simulink model "Simple_4Quad_payload_04"  (R2018b)
settings: Solver=VariableStepAuto  StartTime=0.0  StopTime=60  RelTol=1e-3
InitFcn:
  | Simple_4Quad_payload_04_const
values from neighbouring files (symbols this model uses):
  All_rho = [d1 0 0 ... (first row only)    [Colab_4Quad_model_01_const.m]    (also in Colab_4Quad_model_02_const.m; Simple_4Quad_payload_04_const.m; Simple_4Quad_payload_05_const.m; Simple_4Quad_payload_06_const.m)
  B_ob = [zeros(3);eye(3)]    [Simple_4Quad_payload_04_const.m]    (also in Simple_4Quad_payload_05_const.m; Simple_4Quad_payload_06_const.m; Simple_4Quad_payload_07_const.m; Simple_4Quad_payload_08_const.m)
  BBT_inv = ((B'*B)^(-1))*B'    [Simple_2Quad_payload_03_const.m]    (also in Simple_4Quad_payload_04_const.m = ((BR'*BR)^(-1))*BR'; Simple_4Quad_payload_05_const.m = ((BR'*BR)^(-1))*BR'; Simple_4Quad_payload_06_const.m = ((BR'*BR)^(-1))*BR'; Simple_4Quad_payload_07_const.m = ((BR'*BR)^(-1))*BR')
  BR = 1e0*eye(n)    [Simple_4Quad_payload_04_const.m]    (also in Simple_4Quad_payload_05_const.m; Simple_4Quad_payload_06_const.m; Simple_4Quad_payload_07_const.m; Simple_4Quad_payload_08_const.m)
  C_ob = [eye(3) zeros(3)]    [Simple_4Quad_payload_04_const.m]    (also in Simple_4Quad_payload_05_const.m; Simple_4Quad_payload_06_const.m; Simple_4Quad_payload_07_const.m; Simple_4Quad_payload_08_const.m)
  d1 = 0.25    [Colab_4Quad_model_01_const.m]    (also in Colab_4Quad_model_02_const.m = 0.5; Simple_4Quad_payload_01_const.m = 1; Simple_4Quad_payload_02_const.m = 1; Simple_4Quad_payload_03_const.m = 1)
  d2 = 0.25    [Colab_4Quad_model_01_const.m]    (also in Colab_4Quad_model_02_const.m = 0.5; Simple_4Quad_payload_01_const.m = 1; Simple_4Quad_payload_02_const.m = 1; Simple_4Quad_payload_03_const.m = 1)
  Des_rel_dist = 2    [Simple_4Quad_payload_01_const.m]    (also in Simple_4Quad_payload_02_const.m = 4; Simple_4Quad_payload_03_const.m = 4; Simple_4Quad_payload_04_const.m; Simple_4Quad_payload_05_const.m)
  g = 9.81    [Colab_4Quad_model_01_const.m]    (also in Colab_4Quad_model_02_const.m; Simple_2Quad_payload_01_const.m; Simple_2Quad_payload_02_const.m; Simple_2Quad_payload_03_const.m)
  gamma_0 = 1e-0*diag([1e-3;1e-0])    [Simple_2Quad_payload_03_const.m]    (also in Simple_4Quad_payload_04_const.m = 1e-0*diag([1e-6*ones(3,1);1e-0*ones(3,1)]); Simple_4Quad_payload_05_const.m = 1e-1*diag([1e-6*ones(3,1);1e-0*ones(3,1)]); Simple_4Quad_payload_06_const.m = 1e-0*diag([1e-6*ones(3,1);1e-0*ones(3,1)]); Simple_4Quad_payload_07_const.m = 1e-0*diag([1e-6*ones(3,1);1e-0*ones(3,1)]))
  gamma_1 = 1e+2*diag([1e-3;1e-0])    [Simple_2Quad_payload_03_const.m]    (also in Simple_4Quad_payload_04_const.m = 1e+2*diag([1e-6*ones(3,1);1e-0*ones(3,1)]); Simple_4Quad_payload_05_const.m = 1e+2*diag([1e-6*ones(3,1);1e-0*ones(3,1)]); Simple_4Quad_payload_06_const.m = 1e+3*diag([1e-6*ones(3,1);1e-0*ones(3,1)]); Simple_4Quad_payload_07_const.m = 1e+3*diag([1e-6*ones(3,1);1e-0*ones(3,1)]))
  Ix = 0.166667    [Colab_4Quad_model_01_const.m]    (also in Colab_4Quad_model_02_const.m = 0.02; Simple_4Quad_payload_01_const.m = 1; Simple_4Quad_payload_02_const.m = 1; Simple_4Quad_payload_03_const.m = 1)
  Iy = 0.166667    [Colab_4Quad_model_01_const.m]    (also in Colab_4Quad_model_02_const.m = 0.02; Simple_4Quad_payload_01_const.m = 1; Simple_4Quad_payload_02_const.m = 1; Simple_4Quad_payload_03_const.m = 1)
  Iz = 0.166667    [Colab_4Quad_model_01_const.m]    (also in Colab_4Quad_model_02_const.m = 0.02; Simple_4Quad_payload_01_const.m = 1; Simple_4Quad_payload_02_const.m = 1; Simple_4Quad_payload_03_const.m = 1)
  Jo = diag([Ix;Iy;Iz])    [Colab_4Quad_model_01_const.m]    (also in Colab_4Quad_model_02_const.m; Simple_4Quad_payload_04_const.m; Simple_4Quad_payload_05_const.m; Simple_4Quad_payload_06_const.m)
  Jq = diag([0.0291 0.0291 0.0552])    [Colab_4Quad_model_01_const.m]    (also in Colab_4Quad_model_02_const.m = diag([0.03 0.03 0.06]); Simple_4Quad_payload_03_const.m = 1.2416e-3 * diag([1 1 2]); Simple_4Quad_payload_04_const.m = 1 * diag([1 1 2]); Simple_4Quad_payload_05_const.m = 1 * diag([1 1 2]))
  k1 = 1    [Simple_2Quad_payload_03_const.m]    (also in Simple_4Quad_payload_04_const.m; Simple_4Quad_payload_05_const.m; Simple_4Quad_payload_06_const.m; Simple_4Quad_payload_07_const.m)
  k2 = 0.1    [Simple_2Quad_payload_03_const.m]    (also in Simple_4Quad_payload_04_const.m; Simple_4Quad_payload_05_const.m; Simple_4Quad_payload_06_const.m; Simple_4Quad_payload_07_const.m)
  ki1_N = 0    [Simple_4Quad_payload_02_const.m]    (also in Simple_4Quad_payload_03_const.m; Simple_4Quad_payload_04_const.m; Simple_4Quad_payload_05_const.m; Simple_4Quad_payload_06_const.m)
  ki1_S = 0    [Simple_4Quad_payload_02_const.m]    (also in Simple_4Quad_payload_03_const.m; Simple_4Quad_payload_04_const.m)
  ki2_N = 0    [Simple_4Quad_payload_02_const.m]    (also in Simple_4Quad_payload_03_const.m; Simple_4Quad_payload_04_const.m; Simple_4Quad_payload_05_const.m; Simple_4Quad_payload_06_const.m = 10)
  ki2_S = 0    [Simple_4Quad_payload_02_const.m]    (also in Simple_4Quad_payload_03_const.m; Simple_4Quad_payload_04_const.m)
  kp1_N = 10    [Simple_4Quad_payload_02_const.m]    (also in Simple_4Quad_payload_03_const.m; Simple_4Quad_payload_04_const.m; Simple_4Quad_payload_05_const.m = 1; Simple_4Quad_payload_06_const.m = 1)
  kp1_S = 10    [Simple_4Quad_payload_02_const.m]    (also in Simple_4Quad_payload_03_const.m; Simple_4Quad_payload_04_const.m)
  kp2_N = 100    [Simple_4Quad_payload_02_const.m]    (also in Simple_4Quad_payload_03_const.m; Simple_4Quad_payload_04_const.m; Simple_4Quad_payload_05_const.m = 1; Simple_4Quad_payload_06_const.m = 1)
  kp2_S = 100    [Simple_4Quad_payload_02_const.m]    (also in Simple_4Quad_payload_03_const.m; Simple_4Quad_payload_04_const.m)
  l = 3.1819    [Colab_4Quad_model_01_const.m]    (also in Colab_4Quad_model_02_const.m = 3; Simple_2Quad_payload_04_const.m = 1; Simple_4Quad_payload_01_const.m = 1; Simple_4Quad_payload_02_const.m = 2)
  m = 1.5    [Colab_4Quad_model_01_const.m]    (also in Colab_4Quad_model_02_const.m; Simple_2Quad_payload_04_const.m = 1; Simple_4Quad_payload_01_const.m = 1; Simple_4Quad_payload_02_const.m = 1)
  M = 1.0    (= 1)    [Colab_4Quad_model_01_const.m]    (also in Colab_4Quad_model_02_const.m; Simple_2Quad_payload_01_const.m; Simple_2Quad_payload_02_const.m; Simple_2Quad_payload_03_const.m)
  Md = 1*[1;1;1]    [Simple_2Quad_payload_04_const.m]    (also in Simple_4Quad_payload_01_const.m = 1*[1;1;1;1;1;1]; Simple_4Quad_payload_02_const.m = 1*[1;1;1;1;1;1]; Simple_4Quad_payload_03_const.m = 1*[1;1;1;1;1;1]; Simple_4Quad_payload_04_const.m = 1*[1;1;1;1;1;1])
  n = 2    [Simple_2Quad_payload_03_const.m]    (also in Simple_4Quad_payload_03_const.m = 6; Simple_4Quad_payload_04_const.m = 6; Simple_4Quad_payload_05_const.m = 6; Simple_4Quad_payload_06_const.m = 6)
  Q_ob = var_u_ob * eye(6)    [Simple_4Quad_payload_04_const.m]    (also in Simple_4Quad_payload_05_const.m; Simple_4Quad_payload_06_const.m; Simple_4Quad_payload_07_const.m; Simple_4Quad_payload_08_const.m)
  QR = 1e-0*eye(n)    [Simple_4Quad_payload_04_const.m]    (also in Simple_4Quad_payload_05_const.m = 1e-1*eye(n); Simple_4Quad_payload_06_const.m; Simple_4Quad_payload_07_const.m; Simple_4Quad_payload_08_const.m)
  R = 1e+0*eye(n)    [Simple_2Quad_payload_03_const.m]    (also in Simple_4Quad_payload_04_const.m = 1e+0*eye(m); Simple_4Quad_payload_05_const.m = 1e+0*eye(m); Simple_4Quad_payload_06_const.m; Simple_4Quad_payload_07_const.m)
  R_ob = var_y_ob * eye(3)    [Simple_4Quad_payload_04_const.m]    (also in Simple_4Quad_payload_05_const.m; Simple_4Quad_payload_06_const.m; Simple_4Quad_payload_07_const.m; Simple_4Quad_payload_08_const.m)
  rho_0 = 1e-0    (= 1)    [Simple_2Quad_payload_03_const.m]    (also in Simple_4Quad_payload_04_const.m; Simple_4Quad_payload_05_const.m = 0.1; Simple_4Quad_payload_06_const.m; Simple_4Quad_payload_07_const.m)
  rho_1 = 1e-0    (= 1)    [Simple_2Quad_payload_03_const.m]    (also in Simple_4Quad_payload_04_const.m; Simple_4Quad_payload_05_const.m; Simple_4Quad_payload_06_const.m; Simple_4Quad_payload_07_const.m)
libraries: simulink x16
(part 3 of 4)

== system Simple_4Quad_payload_04/Controllers and Observers/Cotnroller and Observer - Agent1 /PID_alpha1 ==
  alpha1_des : Inport
  alpha1 : Inport  Port=2
  D_alpha1 : Inport  Port=3
  PID Controller : simulink/Continuous/PID Controller  Controller=PID  Form=Parallel  TimeDomain=Continuous-time  SampleTime=-1  IntegratorMethod=Forward Euler  FilterMethod=Forward Euler  ControllerParametersSource=internal  P=kp1_N  I=ki1_N  D=0  UseFilter=on  N=100  TunerSelectOption=Transfer Function Based (PID Tuner App)  InitialConditionSource=internal  InitialConditionForIntegrator=0  InitialConditionForFilter=0  DifferentiatorICPrevScaledInput=0  ExternalReset=none  TrackingMode=off  Kt=1  LimitOutput=off  UpperSaturationLimit=inf  LowerSaturationLimit=-inf  LinearizeAsGain=on  AntiWindupMode=none  Kb=1  POutMin=[]  POutMax=[]  IOutMin=[]  IOutMax=[]  DOutMin=[]  DOutMax=[]  NOutMin=[]  NOutMax=[]  SumOutMin=[]  SumOutMax=[]  SaturationOutMin=[]  SaturationOutMax=[]  PParamMin=[]  PParamMax=[]  IParamMin=[]  IParamMax=[]  DParamMin=[]  DParamMax=[]  NParamMin=[]  NParamMax=[]  KbParamMin=[]  KbParamMax=[]  KtParamMin=[]  KtParamMax=[]  KbOutMin=[]  KbOutMax=[]  KtOutMin=[]  KtOutMax=[]  IntegratorOutMin=[]  IntegratorOutMax=[]  FilterOutMin=[]  FilterOutMax=[]  SumI1OutMin=[]  SumI1OutMax=[]  SumI2OutMin=[]  SumI2OutMax=[]  SumI3OutMin=[]  SumI3OutMax=[]  SumI4OutMin=[]  SumI4OutMax=[]  SumDOutMin=[]  SumDOutMax=[]  DifferentiatorOutMin=[]  DifferentiatorOutMax=[]  FilterDiffOutCoefMin=[]  FilterDiffOutCoefMax=[]  ReciprocalOutMin=[]  ReciprocalOutMax=[]  SumDenOutMin=[]  SumDenOutMax=[]  SumNumOutMin=[]  SumNumOutMax=[]  DivideOutMin=[]  DivideOutMax=[]  IntegratorContinuousStateAttributes=''  IntegratorStateMustResolveToSignalObject=off  IntegratorRTWStateStorageClass=Auto  FilterContinuousStateAttributes=''  FilterStateMustResolveToSignalObject=off  FilterRTWStateStorageClass=Auto  ParallelPVariant=InternalParameters  IdealPVariant=Disabled  IVariant=InternalParameters  DVariant=InternalParameters  IntegratorVariant=Continuous  SatVariant=Disabled  AWVariant=Passthrough  PCopyVariant=Disabled  TRVariant=Disabled  FdbkBlocksVariant=Forward  IdealPFdbkVariant=Disabled  SatFdbkVariant=Disabled  DerivativeFilterVariant=ContFilter  NVariant=InternalParameters  NCopyVariant=Disabled  FilterICVariant=InternalICsFilter  IntegratorICVariant=InternalICs  ExternalResetVariant=Disabled  TRSumVariant=Passthrough  SumFdbkVariant=Disabled  SumVariant=Sum_PID
  PID Controller1 : simulink/Continuous/PID Controller  Controller=PID  Form=Parallel  TimeDomain=Continuous-time  SampleTime=-1  IntegratorMethod=Forward Euler  FilterMethod=Forward Euler  ControllerParametersSource=internal  P=kp2_N  I=ki2_N  D=0  UseFilter=on  N=100  TunerSelectOption=Transfer Function Based (PID Tuner App)  InitialConditionSource=internal  InitialConditionForIntegrator=0  InitialConditionForFilter=0  DifferentiatorICPrevScaledInput=0  ExternalReset=none  TrackingMode=off  Kt=1  LimitOutput=off  UpperSaturationLimit=inf  LowerSaturationLimit=-inf  LinearizeAsGain=on  AntiWindupMode=none  Kb=1  POutMin=[]  POutMax=[]  IOutMin=[]  IOutMax=[]  DOutMin=[]  DOutMax=[]  NOutMin=[]  NOutMax=[]  SumOutMin=[]  SumOutMax=[]  SaturationOutMin=[]  SaturationOutMax=[]  PParamMin=[]  PParamMax=[]  IParamMin=[]  IParamMax=[]  DParamMin=[]  DParamMax=[]  NParamMin=[]  NParamMax=[]  KbParamMin=[]  KbParamMax=[]  KtParamMin=[]  KtParamMax=[]  KbOutMin=[]  KbOutMax=[]  KtOutMin=[]  KtOutMax=[]  IntegratorOutMin=[]  IntegratorOutMax=[]  FilterOutMin=[]  FilterOutMax=[]  SumI1OutMin=[]  SumI1OutMax=[]  SumI2OutMin=[]  SumI2OutMax=[]  SumI3OutMin=[]  SumI3OutMax=[]  SumI4OutMin=[]  SumI4OutMax=[]  SumDOutMin=[]  SumDOutMax=[]  DifferentiatorOutMin=[]  DifferentiatorOutMax=[]  FilterDiffOutCoefMin=[]  FilterDiffOutCoefMax=[]  ReciprocalOutMin=[]  ReciprocalOutMax=[]  SumDenOutMin=[]  SumDenOutMax=[]  SumNumOutMin=[]  SumNumOutMax=[]  DivideOutMin=[]  DivideOutMax=[]  IntegratorContinuousStateAttributes=''  IntegratorStateMustResolveToSignalObject=off  IntegratorRTWStateStorageClass=Auto  FilterContinuousStateAttributes=''  FilterStateMustResolveToSignalObject=off  FilterRTWStateStorageClass=Auto  ParallelPVariant=InternalParameters  IdealPVariant=Disabled  IVariant=InternalParameters  DVariant=InternalParameters  IntegratorVariant=Continuous  SatVariant=Disabled  AWVariant=Passthrough  PCopyVariant=Disabled  TRVariant=Disabled  FdbkBlocksVariant=Forward  IdealPFdbkVariant=Disabled  SatFdbkVariant=Disabled  DerivativeFilterVariant=ContFilter  NVariant=InternalParameters  NCopyVariant=Disabled  FilterICVariant=InternalICsFilter  IntegratorICVariant=InternalICs  ExternalResetVariant=Disabled  TRSumVariant=Passthrough  SumFdbkVariant=Disabled  SumVariant=Sum_PID
  Scope3 : Scope  NumInputPorts=3
  Sum : Sum  Inputs=|+-
  Sum1 : Sum  Inputs=|+-
  N1 : Outport
  wires:
  D_alpha1/1 -> Sum1/2
  alpha1/1 -> Sum/2
  alpha1_des/1 -> Sum/1
  Sum1/1 -> Scope3/2, PID Controller1/1
  Sum/1 -> PID Controller/1, Scope3/1
  PID Controller1/1 -> Scope3/3, N1/1
  PID Controller/1 -> Sum1/1

== system Simple_4Quad_payload_04/Controllers and Observers/Cotnroller and Observer - Agent1 /PID_beta1 ==
  beta1_des : Inport
  beta1 : Inport  Port=2
  D_beta1 : Inport  Port=3
  PID Controller : simulink/Continuous/PID Controller  Controller=PID  Form=Parallel  TimeDomain=Continuous-time  SampleTime=-1  IntegratorMethod=Forward Euler  FilterMethod=Forward Euler  ControllerParametersSource=internal  P=kp1_S  I=ki1_S  D=0  UseFilter=on  N=100  TunerSelectOption=Transfer Function Based (PID Tuner App)  InitialConditionSource=internal  InitialConditionForIntegrator=0  InitialConditionForFilter=0  DifferentiatorICPrevScaledInput=0  ExternalReset=none  TrackingMode=off  Kt=1  LimitOutput=off  UpperSaturationLimit=inf  LowerSaturationLimit=-inf  LinearizeAsGain=on  AntiWindupMode=none  Kb=1  POutMin=[]  POutMax=[]  IOutMin=[]  IOutMax=[]  DOutMin=[]  DOutMax=[]  NOutMin=[]  NOutMax=[]  SumOutMin=[]  SumOutMax=[]  SaturationOutMin=[]  SaturationOutMax=[]  PParamMin=[]  PParamMax=[]  IParamMin=[]  IParamMax=[]  DParamMin=[]  DParamMax=[]  NParamMin=[]  NParamMax=[]  KbParamMin=[]  KbParamMax=[]  KtParamMin=[]  KtParamMax=[]  KbOutMin=[]  KbOutMax=[]  KtOutMin=[]  KtOutMax=[]  IntegratorOutMin=[]  IntegratorOutMax=[]  FilterOutMin=[]  FilterOutMax=[]  SumI1OutMin=[]  SumI1OutMax=[]  SumI2OutMin=[]  SumI2OutMax=[]  SumI3OutMin=[]  SumI3OutMax=[]  SumI4OutMin=[]  SumI4OutMax=[]  SumDOutMin=[]  SumDOutMax=[]  DifferentiatorOutMin=[]  DifferentiatorOutMax=[]  FilterDiffOutCoefMin=[]  FilterDiffOutCoefMax=[]  ReciprocalOutMin=[]  ReciprocalOutMax=[]  SumDenOutMin=[]  SumDenOutMax=[]  SumNumOutMin=[]  SumNumOutMax=[]  DivideOutMin=[]  DivideOutMax=[]  IntegratorContinuousStateAttributes=''  IntegratorStateMustResolveToSignalObject=off  IntegratorRTWStateStorageClass=Auto  FilterContinuousStateAttributes=''  FilterStateMustResolveToSignalObject=off  FilterRTWStateStorageClass=Auto  ParallelPVariant=InternalParameters  IdealPVariant=Disabled  IVariant=InternalParameters  DVariant=InternalParameters  IntegratorVariant=Continuous  SatVariant=Disabled  AWVariant=Passthrough  PCopyVariant=Disabled  TRVariant=Disabled  FdbkBlocksVariant=Forward  IdealPFdbkVariant=Disabled  SatFdbkVariant=Disabled  DerivativeFilterVariant=ContFilter  NVariant=InternalParameters  NCopyVariant=Disabled  FilterICVariant=InternalICsFilter  IntegratorICVariant=InternalICs  ExternalResetVariant=Disabled  TRSumVariant=Passthrough  SumFdbkVariant=Disabled  SumVariant=Sum_PID
  PID Controller1 : simulink/Continuous/PID Controller  Controller=PID  Form=Parallel  TimeDomain=Continuous-time  SampleTime=-1  IntegratorMethod=Forward Euler  FilterMethod=Forward Euler  ControllerParametersSource=internal  P=kp2_S  I=ki2_S  D=0  UseFilter=on  N=100  TunerSelectOption=Transfer Function Based (PID Tuner App)  InitialConditionSource=internal  InitialConditionForIntegrator=0  InitialConditionForFilter=0  DifferentiatorICPrevScaledInput=0  ExternalReset=none  TrackingMode=off  Kt=1  LimitOutput=off  UpperSaturationLimit=inf  LowerSaturationLimit=-inf  LinearizeAsGain=on  AntiWindupMode=none  Kb=1  POutMin=[]  POutMax=[]  IOutMin=[]  IOutMax=[]  DOutMin=[]  DOutMax=[]  NOutMin=[]  NOutMax=[]  SumOutMin=[]  SumOutMax=[]  SaturationOutMin=[]  SaturationOutMax=[]  PParamMin=[]  PParamMax=[]  IParamMin=[]  IParamMax=[]  DParamMin=[]  DParamMax=[]  NParamMin=[]  NParamMax=[]  KbParamMin=[]  KbParamMax=[]  KtParamMin=[]  KtParamMax=[]  KbOutMin=[]  KbOutMax=[]  KtOutMin=[]  KtOutMax=[]  IntegratorOutMin=[]  IntegratorOutMax=[]  FilterOutMin=[]  FilterOutMax=[]  SumI1OutMin=[]  SumI1OutMax=[]  SumI2OutMin=[]  SumI2OutMax=[]  SumI3OutMin=[]  SumI3OutMax=[]  SumI4OutMin=[]  SumI4OutMax=[]  SumDOutMin=[]  SumDOutMax=[]  DifferentiatorOutMin=[]  DifferentiatorOutMax=[]  FilterDiffOutCoefMin=[]  FilterDiffOutCoefMax=[]  ReciprocalOutMin=[]  ReciprocalOutMax=[]  SumDenOutMin=[]  SumDenOutMax=[]  SumNumOutMin=[]  SumNumOutMax=[]  DivideOutMin=[]  DivideOutMax=[]  IntegratorContinuousStateAttributes=''  IntegratorStateMustResolveToSignalObject=off  IntegratorRTWStateStorageClass=Auto  FilterContinuousStateAttributes=''  FilterStateMustResolveToSignalObject=off  FilterRTWStateStorageClass=Auto  ParallelPVariant=InternalParameters  IdealPVariant=Disabled  IVariant=InternalParameters  DVariant=InternalParameters  IntegratorVariant=Continuous  SatVariant=Disabled  AWVariant=Passthrough  PCopyVariant=Disabled  TRVariant=Disabled  FdbkBlocksVariant=Forward  IdealPFdbkVariant=Disabled  SatFdbkVariant=Disabled  DerivativeFilterVariant=ContFilter  NVariant=InternalParameters  NCopyVariant=Disabled  FilterICVariant=InternalICsFilter  IntegratorICVariant=InternalICs  ExternalResetVariant=Disabled  TRSumVariant=Passthrough  SumFdbkVariant=Disabled  SumVariant=Sum_PID
  Scope3 : Scope  NumInputPorts=3
  Sum : Sum  Inputs=|+-
  Sum1 : Sum  Inputs=|+-
  S1 : Outport
  wires:
  D_beta1/1 -> Sum1/2
  PID Controller/1 -> Sum1/1
  PID Controller1/1 -> S1/1, Scope3/3
  Sum/1 -> Scope3/1, PID Controller/1
  Sum1/1 -> PID Controller1/1, Scope3/2
  beta1_des/1 -> Sum/1
  beta1/1 -> Sum/2

== system Simple_4Quad_payload_04/Controllers and Observers/Cotnroller and Observer - Agent1 /Rotation_Q1 ==
  Omega Q1 : Inport
  D Phi : MATLAB Function  TreatAsAtomicUnit=on
  Integrator : Integrator  InitialCondition=zeros(3,1)
  Mux : Mux  Inputs=2
  X_Rot_Q1 : Outport
  wires:
  D Phi/1(D_PHI_Q1) -> Integrator/1
  Omega Q1/1 -> D Phi/1(Omega_Q1), Mux/2
  Integrator/1 -> D Phi/2(PHI_Q1), Mux/1
  Mux/1 -> X_Rot_Q1/1

== system Simple_4Quad_payload_04/Controllers and Observers/Cotnroller and Observer - Agent1 /Rotational #1 ==
  x_rd : Inport
  X : Inport  Port=2
  CARE : MATLAB Function  TreatAsAtomicUnit=on
  Differentiator : Subsystem
  Integrator : Integrator  InitialCondition=zeros(n)
  Integrator1 : Integrator  InitialCondition=eye(n)
  Integrator2 : Integrator  InitialCondition=zeros(n,1)
  Integrator3 : Integrator  InitialCondition=zeros(n,1)
  Memory : Memory  InitialCondition=zeros(n,1)
  Sum : Sum  Inputs=|++
  g-Estimator : MATLAB Function  TreatAsAtomicUnit=on
  g-Estimator1 : MATLAB Function  TreatAsAtomicUnit=on
  main : MATLAB Function  TreatAsAtomicUnit=on
  output definition : MATLAB Function  TreatAsAtomicUnit=on
  variable change : MATLAB Function  TreatAsAtomicUnit=on
  ur1 : Outport
  tag scope: A_hat1_R=global, P1_R=global, e1_R=global, g_hat1_R=global
  wires:
  x_rd/1 -> variable change/2(Xd)
  X/1 -> variable change/1(X)
  CARE/1(DP) -> Integrator1/1
  Sum/1 -> main/1(sigma), g-Estimator/1(sigma), g-Estimator1/1(sigma)
  g-Estimator1/1(Da_hat) -> Integrator/1
  variable change/1(x_mod) -> main/7(x), g-Estimator1/2(x)
  Integrator1/1 -> g-Estimator1/3(P), CARE/1(P), [P1_R], g-Estimator/3(P), main/4(P)
  Integrator/1 -> [A_hat1_R], g-Estimator1/4(a_hat), CARE/2(a_hat), main/5(a_hat)
  g-Estimator/1(Dg_hat) -> Integrator2/1
  Differentiator/1(Dx_d) -> main/3(Dy_d)
  main/1(u) -> output definition/1(u), Memory/1
  Integrator3/1 -> main/2(zeta), Sum/1
  variable change/2(xd_mod) -> Differentiator/1(x_d)
  variable change/3(e_mod) -> [e1_R], Sum/2, Integrator3/1
  Memory/1 -> variable change/3(u)
  Integrator2/1 -> main/6(g_hat), [g_hat1_R], g-Estimator/2(g_hat)
  output definition/1(ur) -> ur1/1

== system Simple_4Quad_payload_04/Controllers and Observers/Controlelr and Observer - Agent3/Rotational #3/Differentiator ==
  x_d : Inport
  Integrator : Integrator  InitialCondition=zeros(n,1)
  Integrator1 : Integrator  InitialCondition=zeros(n,1)
  Scope : Scope
  Scope1 : Scope
  Sliding differentiator : MATLAB Function  TreatAsAtomicUnit=on
  Sliding differentiator1 : MATLAB Function  TreatAsAtomicUnit=on
  Sum : Sum  Inputs=|-+
  Dx_d : Outport
  wires:
  Integrator1/1 -> Sum/2
  Sum/1 -> Sliding differentiator1/1(e), Sliding differentiator/2(e), Scope1/1
  x_d/1 -> Sum/1
  Integrator/1 -> Sliding differentiator/1(u1)
  Sliding differentiator1/1(Du1) -> Integrator/1
  Sliding differentiator/1(u) -> Dx_d/1, Integrator1/1, Scope/1

== system Simple_4Quad_payload_04/Controllers and Observers/Controller and Observer - Agent2/Rotational #2/Differentiator ==
  x_d : Inport
  Integrator : Integrator  InitialCondition=zeros(n,1)
  Integrator1 : Integrator  InitialCondition=zeros(n,1)
  Scope : Scope
  Scope1 : Scope
  Sliding differentiator : MATLAB Function  TreatAsAtomicUnit=on
  Sliding differentiator1 : MATLAB Function  TreatAsAtomicUnit=on
  Sum : Sum  Inputs=|-+
  Dx_d : Outport
  wires:
  Sliding differentiator/1(u) -> Scope/1, Integrator1/1, Dx_d/1
  Sliding differentiator1/1(Du1) -> Integrator/1
  Integrator/1 -> Sliding differentiator/1(u1)
  x_d/1 -> Sum/1
  Sum/1 -> Scope1/1, Sliding differentiator/2(e), Sliding differentiator1/1(e)
  Integrator1/1 -> Sum/2

== system Simple_4Quad_payload_04/Controllers and Observers/Controller and Observer - Agent4/Rotational #4/Differentiator ==
  x_d : Inport
  Integrator : Integrator  InitialCondition=zeros(n,1)
  Integrator1 : Integrator  InitialCondition=zeros(n,1)
  Scope : Scope
  Scope1 : Scope
  Sliding differentiator : MATLAB Function  TreatAsAtomicUnit=on
  Sliding differentiator1 : MATLAB Function  TreatAsAtomicUnit=on
  Sum : Sum  Inputs=|-+
  Dx_d : Outport
  wires:
  Sliding differentiator/1(u) -> Scope/1, Integrator1/1, Dx_d/1
  Sliding differentiator1/1(Du1) -> Integrator/1
  Integrator/1 -> Sliding differentiator/1(u1)
  x_d/1 -> Sum/1
  Sum/1 -> Scope1/1, Sliding differentiator/2(e), Sliding differentiator1/1(e)
  Integrator1/1 -> Sum/2

== system Simple_4Quad_payload_04/Controllers and Observers/Cotnroller and Observer - Agent1 /Rotational #1/Differentiator ==
  x_d : Inport
  Integrator : Integrator  InitialCondition=zeros(n,1)
  Integrator1 : Integrator  InitialCondition=zeros(n,1)
  Sliding differentiator : MATLAB Function  TreatAsAtomicUnit=on
  Sliding differentiator1 : MATLAB Function  TreatAsAtomicUnit=on
  Sum : Sum  Inputs=|-+
  Dx_d : Outport
  wires:
  Sliding differentiator/1(u) -> Integrator1/1, Dx_d/1
  Sliding differentiator1/1(Du1) -> Integrator/1
  Integrator/1 -> Sliding differentiator/1(u1)
  x_d/1 -> Sum/1
  Sum/1 -> Sliding differentiator/2(e), Sliding differentiator1/1(e)
  Integrator1/1 -> Sum/2

== matlab function Simple_4Quad_payload_04/Controllers and Observers/Controller - Payload/Controller ==
  data: e input; F output; Alpha_Des output; PHI input; Beta_Des output; Md parameter; g parameter; M parameter; OUT output; d1 parameter; d2 parameter; Ix parameter; Iy parameter; Iz parameter; l parameter; Des_rel_dist parameter
function [F,Alpha_Des,Beta_Des,OUT] = fcn(e,PHI, Md, g, M, d1, d2, Ix, Iy, Iz, l, Des_rel_dist)

phi = PHI(1);
theta = PHI(2);
psi = PHI(3);

Io = diag([Ix;Iy;Iz]);

Ro = [cos(psi)*cos(theta) cos(psi)*sin(theta)*sin(phi)-sin(psi)*cos(phi) cos(psi)*sin(theta)*cos(phi)+sin(psi)*sin(phi);
    sin(psi)*cos(theta) sin(psi)*sin(theta)*sin(phi)+cos(psi)*cos(phi) sin(psi)*sin(theta)*cos(phi)-cos(psi)*sin(phi);
    -sin(theta) cos(theta)*sin(phi) cos(theta)*cos(phi)];

s1 = [0 0 0;
    0 0 -d1;
    0 d1 0];

s2 = [0 0 0;
    0 0 d1;
    0 -d1 0];

s3 = [0 0 d2;
    0 0 0;
    -d2 0 0];

s4 = [0 0 -d2;
    0 0 0;
    d2 0 0];

B = [(1/M)*Ro (1/M)*Ro (1/M)*Ro (1/M)*Ro;
    Io^(-1)*s1 Io^(-1)*s2 Io^(-1)*s3 Io^(-1)*s4;
    1 0 0 1 0 0 0 0 0 0 0 0;
    0 0 0 0 0 0 0 1 0 0 1 0;
    1 0 0 0 0 0 0 0 0 0 0 0;
    0 0 0 0 0 0 0 1 0 0 0 0];

D = [0;0;-g;0;0;0];

SGN = zeros(6);
for i=1:6
    SGN(i,i) = e(i)/(abs(e(i))+0.1);
end

Z = SGN*Md;
U = Z - D;

u_t = U(1:3);
rx_des = Des_rel_dist;
ry_des = Des_rel_dist;
q1 = (rx_des - (2*d1)) / (2*l);
q2 = (ry_des - (2*d2)) / (2*l);
K1 = sqrt( ((u_t(2)/2)^2 + (u_t(3)/4)^2) / ((1/(q1^2))-1) );
K2 = sqrt( ((u_t(1)/2)^2 + (u_t(3)/4)^2) / ((1/(q2^2))-1) );

U_gen = [U;0;0;K1;K2];

Mu = B' * (B*B')^(-1) * U_gen;

F = zeros(4,1);
Alpha_Des = zeros(4,1);
Beta_Des = zeros(4,1);

for i=1:4
    F(i,1) = sqrt( Mu((3*(i-1)+1):(3*(i-1)+3))'*Mu((3*(i-1)+1):(3*(i-1)+3)) );
    Alpha_Des(i,1) = asin( max(min(Mu(3*(i-1)+3,1)/F(i,1),1),-1) );
    Beta_Des(i,1) = atan2( Mu(3*(i-1)+2,1),Mu(3*(i-1)+1,1) );
    if Beta_Des(i,1) < (-3*pi/4)
        Beta_Des(i,1) = 2*pi + Beta_Des(i,1);
    end
end

OUT = U;

end

== matlab function Simple_4Quad_payload_04/Controllers and Observers/Cotnroller and Observer - Agent1 /Rotation_Q1/D Phi ==
  data: Omega_Q1 input; D_PHI_Q1 output; PHI_Q1 input
function D_PHI_Q1 = fcn(Omega_Q1,PHI_Q1)

phi_q1 = PHI_Q1(1);
theta_q1 = PHI_Q1(2);

Rm_Q1 = [1 0 -sin(theta_q1);
    0 cos(phi_q1) cos(theta_q1)*sin(phi_q1);
    0 -sin(phi_q1) cos(theta_q1)*cos(phi_q1)];

D_PHI_Q1 = (Rm_Q1)^(-1) * Omega_Q1;


end

== matlab function Simple_4Quad_payload_04/Controllers and Observers/Controller and Observer - Agent2/Dynamic Model2 ==
  data: N2 input; S2 input; f2 input; alpha2 input; beta2 input; D_alpha2 input; D_beta2 input; m parameter; g parameter; DD_PHI input; DD_P input; D_PHI input; l parameter; d1 parameter; PHI input; U2_local output; U2 output
function [U2_local,U2]  = fcn(N2,S2,f2,alpha2,beta2,D_alpha2,D_beta2,m, g,DD_PHI,DD_P,D_PHI, l, d1,PHI)

phi = PHI(1);
theta = PHI(2);
psi = PHI(3);

Dist2_local = [-d1;0;0];
D2_angles = [0;D_alpha2;D_beta2];

Ro = [cos(psi)*cos(theta) cos(psi)*sin(theta)*sin(phi)-sin(psi)*cos(phi) cos(psi)*sin(theta)*cos(phi)+sin(psi)*sin(phi);
    sin(psi)*cos(theta) sin(psi)*sin(theta)*sin(phi)+cos(psi)*cos(phi) sin(psi)*sin(theta)*cos(phi)-cos(psi)*sin(phi);
    -sin(theta) cos(theta)*sin(phi) cos(theta)*cos(phi)];

R2 = [cos(alpha2)*cos(beta2) -sin(beta2) -sin(alpha2)*cos(beta2);
    cos(alpha2)*sin(beta2) cos(beta2) -sin(alpha2)*sin(beta2);
    sin(alpha2) 0 cos(alpha2)];

C1_2 = External_Product3(D_PHI,Dist2_local);
C2_2 = External_Product3(D_PHI,C1_2);
C3_2 = External_Product3(DD_PHI,Dist2_local);

C4_2 = External_Product3(D2_angles,Dist2_local);
C5_2 = External_Product3(D2_angles,C4_2);

a2_part = (  R2' * ( Ro'*DD_P + C2_2 + C3_2 ) ) + C5_2;

G2_local = R2' * Ro' * [0;0;-g];

T2 = m*a2_part(1) + f2 - m*G2_local(1);
%DD_alpha2 = (1/m/l) * (N2 - m*a2_part(2) + m*G2_local(2));
%DD_beta2 = (1/m/l) * (S2 - m*a2_part(3) + m*G2_local(3));

U2_local = [f2+m*g;0;0;]; % [T2;S2;N2];

U2 = Ro * R2 * U2_local;

end

== matlab function Simple_4Quad_payload_04/Controllers and Observers/Cotnroller and Observer - Agent1 /Dynamic Model1 ==
  data: N1 input; S1 input; f1 input; alpha1 input; beta1 input; D_alpha1 input; D_beta1 input; m parameter; g parameter; DD_PHI input; DD_P input; D_PHI input; l parameter; d1 parameter; PHI input; U1_local output; U1 output
function [U1_local,U1]  = fcn(N1,S1,f1,alpha1,beta1,D_alpha1,D_beta1,m, g,DD_PHI,DD_P,D_PHI, l, d1,PHI)

phi = PHI(1);
theta = PHI(2);
psi = PHI(3);

Dist1_local = [d1;0;0];
D1_angles = [0;D_alpha1;D_beta1];

Ro = [cos(psi)*cos(theta) cos(psi)*sin(theta)*sin(phi)-sin(psi)*cos(phi) cos(psi)*sin(theta)*cos(phi)+sin(psi)*sin(phi);
    sin(psi)*cos(theta) sin(psi)*sin(theta)*sin(phi)+cos(psi)*cos(phi) sin(psi)*sin(theta)*cos(phi)-cos(psi)*sin(phi);
    -sin(theta) cos(theta)*sin(phi) cos(theta)*cos(phi)];

R1 = [cos(alpha1)*cos(beta1) -sin(beta1) -sin(alpha1)*cos(beta1);
    cos(alpha1)*sin(beta1) cos(beta1) -sin(alpha1)*sin(beta1);
    sin(alpha1) 0 cos(alpha1)];

C1_1 = External_Product3(D_PHI,Dist1_local);
C2_1 = External_Product3(D_PHI,C1_1);
C3_1 = External_Product3(DD_PHI,Dist1_local);

C4_1 = External_Product3(D1_angles,Dist1_local);
C5_1 = External_Product3(D1_angles,C4_1);

a1_part = (  R1' * ( Ro'*DD_P + C2_1 + C3_1 ) ) + C5_1;

G1_local = R1' * Ro' * [0;0;-g];

T1 = m*a1_part(1) + f1 - m*G1_local(1);
%DD_alpha1 = (1/m/l) * (N1 - m*a1_part(2) + m*G1_local(2));
%DD_beta1 = (1/m/l) * (S1 - m*a1_part(3) + m*G1_local(3));

U1_local = [f1+m*g;0;0;]; % [T1;S1;N1];

U1 = Ro * R1 * U1_local;

end

== matlab function Simple_4Quad_payload_04/Controllers and Observers/Controller and Observer - Agent4/Dynamic Model4 ==
  data: N4 input; S4 input; f4 input; alpha4 input; beta4 input; D_alpha4 input; D_beta4 input; m parameter; g parameter; DD_PHI input; DD_P input; D_PHI input; l parameter; d2 parameter; PHI input; U4_local output; U4 output
function [U4_local,U4]  = fcn(N4,S4,f4,alpha4,beta4,D_alpha4,D_beta4,m, g,DD_PHI,DD_P,D_PHI, l, d2,PHI)

phi = PHI(1);
theta = PHI(2);
psi = PHI(3);

Dist4_local = [0;-d2;0];
D4_angles = [0;D_alpha4;D_beta4];

Ro = [cos(psi)*cos(theta) cos(psi)*sin(theta)*sin(phi)-sin(psi)*cos(phi) cos(psi)*sin(theta)*cos(phi)+sin(psi)*sin(phi);
    sin(psi)*cos(theta) sin(psi)*sin(theta)*sin(phi)+cos(psi)*cos(phi) sin(psi)*sin(theta)*cos(phi)-cos(psi)*sin(phi);
    -sin(theta) cos(theta)*sin(phi) cos(theta)*cos(phi)];

R4 = [cos(alpha4)*cos(beta4) -sin(beta4) -sin(alpha4)*cos(beta4);
    cos(alpha4)*sin(beta4) cos(beta4) -sin(alpha4)*sin(beta4);
    sin(alpha4) 0 cos(alpha4)];

C1_4 = External_Product3(D_PHI,Dist4_local);
C2_4 = External_Product3(D_PHI,C1_4);
C3_4 = External_Product3(DD_PHI,Dist4_local);

C4_4 = External_Product3(D4_angles,Dist4_local);
C5_4 = External_Product3(D4_angles,C4_4);

a4_part = (  R4' * ( Ro'*DD_P + C2_4 + C3_4 ) ) + C5_4;

G4_local = R4' * Ro' * [0;0;-g];

T4 = m*a4_part(1) + f4 - m*G4_local(1);
%DD_alpha4 = (1/m/l) * (N4 - m*a4_part(2) + m*G4_local(2));
%DD_beta4 = (1/m/l) * (S4 - m*a4_part(3) + m*G4_local(3));

U4_local = [f4+m*g;0;0;]; % [T4;S4;N4];

U4 = Ro * R4 * U4_local;

end

== matlab function Simple_4Quad_payload_04/Controllers and Observers/Controlelr and Observer - Agent3/Dynamic Model3 ==
  data: N3 input; S3 input; f3 input; alpha3 input; beta3 input; D_alpha3 input; D_beta3 input; m parameter; g parameter; DD_PHI input; DD_P input; D_PHI input; l parameter; d2 parameter; PHI input; U3_local output; U3 output
function [U3_local,U3]  = fcn(N3,S3,f3,alpha3,beta3,D_alpha3,D_beta3,m, g,DD_PHI,DD_P,D_PHI, l, d2,PHI)

phi = PHI(1);
theta = PHI(2);
psi = PHI(3);

Dist3_local = [0;d2;0];
D3_angles = [0;D_alpha3;D_beta3];

Ro = [cos(psi)*cos(theta) cos(psi)*sin(theta)*sin(phi)-sin(psi)*cos(phi) cos(psi)*sin(theta)*cos(phi)+sin(psi)*sin(phi);
    sin(psi)*cos(theta) sin(psi)*sin(theta)*sin(phi)+cos(psi)*cos(phi) sin(psi)*sin(theta)*cos(phi)-cos(psi)*sin(phi);
    -sin(theta) cos(theta)*sin(phi) cos(theta)*cos(phi)];

R3 = [cos(alpha3)*cos(beta3) -sin(beta3) -sin(alpha3)*cos(beta3);
    cos(alpha3)*sin(beta3) cos(beta3) -sin(alpha3)*sin(beta3);
    sin(alpha3) 0 cos(alpha3)];

C1_3 = External_Product3(D_PHI,Dist3_local);
C2_3 = External_Product3(D_PHI,C1_3);
C3_3 = External_Product3(DD_PHI,Dist3_local);

C4_3 = External_Product3(D3_angles,Dist3_local);
C5_3 = External_Product3(D3_angles,C4_3);

a3_part = (  R3' * ( Ro'*DD_P + C2_3 + C3_3 ) ) + C5_3;

G3_local = R3' * Ro' * [0;0;-g];

T3 = m*a3_part(1) + f3 - m*G3_local(1);
%DD_alpha3 = (1/m/l) * (N3 - m*a3_part(2) + m*G3_local(2));
%DD_beta3 = (1/m/l) * (S3 - m*a3_part(3) + m*G3_local(3));

U3_local = [f3+m*g;0;0;]; % [T3;S3;N3];

U3 = Ro * R3 * U3_local;

end

== matlab function Simple_4Quad_payload_04/Relative Positions scopes/MATLAB Function ==
  data: P1 input; e_cons_1 output; P2 input; P3 input; P4 input; e_cons_2 output; e_cons_3 output; e_cons_4 output; Des_rel_dist parameter
function [e_cons_1,e_cons_2,e_cons_3,e_cons_4] = fcn(P1,P2,P3,P4,Des_rel_dist)

Pos_local_1 = [Des_rel_dist/2;0;0];
Pos_local_2 = [-Des_rel_dist/2;0;0];
Pos_local_3 = [0;Des_rel_dist/2;0];
Pos_local_4 = [0;-Des_rel_dist/2;0];

Pos_All = [P1 P2 P3 P4];
Pos_local_All = [Pos_local_1 Pos_local_2 Pos_local_3 Pos_local_4];
e_cons_All = zeros(3,4);

for i=1:4
    for j=1:4
        e_cons_All(:,i) = e_cons_All(:,i) + ( (Pos_All(:,i)-Pos_All(:,j)) - (Pos_local_All(:,i)-Pos_local_All(:,j)) );
    end
end

e_cons_1 = e_cons_All(:,1);
e_cons_2 = e_cons_All(:,2);
e_cons_3 = e_cons_All(:,3);
e_cons_4 = e_cons_All(:,4);

end

== matlab function Simple_4Quad_payload_04/Controllers and Observers/Controller - Payload/MATLAB Function ==
  data: t input; Vd output
function Vd = fcn(t)

fv = 0.2;
rv = 1;
Vdz = 0.2;
Vd = [rv*fv*sin(fv*t);
    -rv*fv*cos(fv*t);
    Vdz];

end

== matlab function Simple_4Quad_payload_04/Dynamic model of the entire system/Dynamic Model  ==
  data: DD_PHI output; D_PHI output; D_Omegao output; D_omegai_1 output; D_omegai_2 output; D_omegai_3 output; D_omegai_4 output; D_Omega_Q1 output; D_Omega_Q2 output; D_Omega_Q3 output; D_Omega_Q4 output; Dq1 output; Dq2 output; Dq3 output; Dq4 output; DDq1 output; DDq2 output; DDq3 output; DDq4 output; alphas input; betas input; PHI input; Omegao input; omegai1 input; omegai2 input; omegai3 input; omegai4 input; Omega_q1 input; Omega_q2 input; Omega_q3 input; Omega_q4 input; q1 input; q2 input; q3 input; q4 input; DD_Po output; d2 parameter; M parameter; Jo parameter; g parameter; d1 parameter; m parameter; l parameter; Tau_q1 input; Tau_q2 input; Tau_q3 input; Tau_q4 input; Jq parameter; U1_local input; U2_local input; U3_local input; U4_local input
function [DD_PHI,D_PHI,D_Omegao,D_omegai_1,D_omegai_2,D_omegai_3,D_omegai_4,D_Omega_Q1,D_Omega_Q2,D_Omega_Q3,D_Omega_Q4,Dq1,Dq2,Dq3,Dq4,DDq1,DDq2,DDq3,DDq4,DD_Po] = ...
    fcn(alphas,betas,PHI,Omegao,omegai1,omegai2,omegai3,omegai4,Omega_q1,Omega_q2,Omega_q3,Omega_q4,q1,q2,q3,q4,d2, M,Jo,g, d1, m, l,Tau_q1,Tau_q2,Tau_q3,Tau_q4, Jq, U1_local,U2_local,U3_local,U4_local)

alpha1 = alphas(1);
alpha2 = alphas(2);
alpha3 = alphas(3);
alpha4 = alphas(4);

beta1 = betas(1);
beta2 = betas(2);
beta3 = betas(3);
beta4 = betas(4);

phi = PHI(1);
theta = PHI(2);
psi = PHI(3);

R1 = [cos(alpha1)*cos(beta1) -sin(beta1) -sin(alpha1)*cos(beta1);
    cos(alpha1)*sin(beta1) cos(beta1) -sin(alpha1)*sin(beta1);
    sin(alpha1) 0 cos(alpha1)];

R2 = [cos(alpha2)*cos(beta2) -sin(beta2) -sin(alpha2)*cos(beta2);
    cos(alpha2)*sin(beta2) cos(beta2) -sin(alpha2)*sin(beta2);
    sin(alpha2) 0 cos(alpha2)];

R3 = [cos(alpha3)*cos(beta3) -sin(beta3) -sin(alpha3)*cos(beta3);
    cos(alpha3)*sin(beta3) cos(beta3) -sin(alpha3)*sin(beta3);
    sin(alpha3) 0 cos(alpha3)];

R4 = [cos(alpha4)*cos(beta4) -sin(beta4) -sin(alpha4)*cos(beta4);
    cos(alpha4)*sin(beta4) cos(beta4) -sin(alpha4)*sin(beta4);
    sin(alpha4) 0 cos(alpha4)];

Ro = [cos(psi)*cos(theta) cos(psi)*sin(theta)*sin(phi)-sin(psi)*cos(phi) cos(psi)*sin(theta)*cos(phi)+sin(psi)*sin(phi);
    sin(psi)*cos(theta) sin(psi)*sin(theta)*sin(phi)+cos(psi)*cos(phi) sin(psi)*sin(theta)*cos(phi)-cos(psi)*sin(phi);
    -sin(theta) cos(theta)*sin(phi) cos(theta)*cos(phi)];

r1 = [d1;0;0];
r2 = [-d1;0;0];
r3 = [0;d2;0];
r4 = [0;-d2;0];

G = [0;0;-g];



%% 
Ri = struct('val',repmat({zeros(3)},4,1));
Ui_local = struct('val',repmat({zeros(3,1)},4,1));
ri = struct('val',repmat({zeros(3,1)},4,1));
ri_skew = struct('val',repmat({zeros(3)},4,1));
qi_body = struct('val',repmat({zeros(3,1)},4,1));
qi_inert = struct('val',repmat({zeros(3,1)},4,1));
qi_inert_skew = struct('val',repmat({zeros(3)},4,1));
Mq = struct('val',repmat({zeros(3,1)},4,1));
Omega_Qi_skew = struct('val',repmat({zeros(3)},4,1));
Omega_Qi = struct('val',repmat({zeros(3,1)},4,1));
D_Omega_Qi = struct('val',repmat({zeros(3,1)},4,1));

Ri(1).val = R1;
Ri(2).val = R2;
Ri(3).val = R3;
Ri(4).val = R4;

Ui_local(1).val = U1_local;
Ui_local(2).val = U2_local;
Ui_local(3).val = U3_local;
Ui_local(4).val = U4_local;

ri(1).val = r1;
ri(2).val = r2;
ri(3).val = r3;
ri(4).val = r4;

ri_skew(1).val = ... 
    [0 -r1(3) r1(2);
    r1(3) 0 -r1(1);
    -r1(2) r1(1) 0];

ri_skew(2).val = ... 
    [0 -r2(3) r2(2);
    r2(3) 0 -r2(1);
    -r2(2) r2(1) 0];

ri_skew(3).val = ... 
    [0 -r3(3) r3(2);
    r3(3) 0 -r3(1);
    -r3(2) r3(1) 0];

ri_skew(4).val = ... 
    [0 -r4(3) r4(2);
    r4(3) 0 -r4(1);
    -r4(2) r4(1) 0];

qi_body(1).val = R1 * [1;0;0];
qi_body(2).val = R2 * [1;0;0];
qi_body(3).val = R3 * [1;0;0];
qi_body(4).val = R4 * [1;0;0];

qi_inert(1).val = Ro * qi_body(1).val;
qi_inert(2).val = Ro * qi_body(2).val;
qi_inert(3).val = Ro * qi_body(3).val;
qi_inert(4).val = Ro * qi_body(4).val;

qi_inert_skew(1).val = ...
    [0 -qi_inert(1).val(3) qi_inert(1).val(2);
    qi_inert(1).val(3) 0 -qi_inert(1).val(1);
    -qi_inert(1).val(2) qi_inert(1).val(1) 0];

qi_inert_skew(2).val = ...
    [0 -qi_inert(2).val(3) qi_inert(2).val(2);
    qi_inert(2).val(3) 0 -qi_inert(2).val(1);
    -qi_inert(2).val(2) qi_inert(2).val(1) 0];

qi_inert_skew(3).val = ...
    [0 -qi_inert(3).val(3) qi_inert(3).val(2);
    qi_inert(3).val(3) 0 -qi_inert(3).val(1);
    -qi_inert(3).val(2) qi_inert(3).val(1) 0];

qi_inert_skew(4).val = ...
    [0 -qi_inert(4).val(3) qi_inert(4).val(2);
    qi_inert(4).val(3) 0 -qi_inert(4).val(1);
    -qi_inert(4).val(2) qi_inert(4).val(1) 0];

Omegao_skew = ...
    [0 -Omegao(3) Omegao(2);
    Omegao(3) 0 -Omegao(1);
    -Omegao(2) Omegao(1) 0];

Mag2_omegai = ...
    [omegai1'*omegai1;
    omegai2'*omegai2;
    omegai3'*omegai3;
    omegai4'*omegai4];

Mq(1).val = Tau_q1;
Mq(2).val = Tau_q2;
Mq(3).val = Tau_q3;
Mq(4).val = Tau_q4;

Omega_Qi(1).val = Omega_q1;
Omega_Qi(2).val = Omega_q2;
Omega_Qi(3).val = Omega_q3;
Omega_Qi(4).val = Omega_q4;

Omega_Qi_skew(1).val = ...
    [0 -Omega_Qi(1).val(3) Omega_Qi(1).val(2);
    Omega_Qi(1).val(3) 0 -Omega_Qi(1).val(1);
    -Omega_Qi(1).val(2) Omega_Qi(1).val(1) 0];

Omega_Qi_skew(2).val = ...
    [0 -Omega_Qi(2).val(3) Omega_Qi(2).val(2);
    Omega_Qi(2).val(3) 0 -Omega_Qi(2).val(1);
    -Omega_Qi(2).val(2) Omega_Qi(2).val(1) 0];

Omega_Qi_skew(3).val = ...
    [0 -Omega_Qi(3).val(3) Omega_Qi(3).val(2);
    Omega_Qi(3).val(3) 0 -Omega_Qi(3).val(1);
    -Omega_Qi(3).val(2) Omega_Qi(3).val(1) 0];

Omega_Qi_skew(4).val = ...
    [0 -Omega_Qi(4).val(3) Omega_Qi(4).val(2);
    Omega_Qi(4).val(3) 0 -Omega_Qi(4).val(1);
    -Omega_Qi(4).val(2) Omega_Qi(4).val(1) 0];


%% Dynamics of the entire system
u_DDP = zeros(3,1);
u_DOmega = zeros(3,1);
term_g_DDP = (M*G);
term_DOmega_DDP = zeros(3);
term_Omega2_DDP = zeros(3,1);
term_omegai2_DDP = zeros(3,1);
term_DOmega_DOmega = zeros(3);
term_Omega2_DOmega = zeros(3,1);
term_DDP_DOmega = zeros(3);
term_omegai2_DOmega = zeros(3,1);
term_g_DOmega = zeros(3,1);

M_tot = zeros(18,18);
F_tot = zeros(18,1);

for i=1:4
    u_DDP = u_DDP + ( Ro * Ri(i).val * Ui_local(i).val );
    u_DOmega = u_DOmega + ( ri_skew(i).val * Ri(i).val * Ui_local(i).val );
    term_DOmega_DDP = term_DOmega_DDP + ( m * qi_inert(i).val * qi_inert(i).val' * Ro * ri_skew(i).val );
    term_Omega2_DDP = term_Omega2_DDP + ( m * qi_inert(i).val * qi_inert(i).val' * Ro * Omegao_skew * Omegao_skew * ri(i).val );
    term_omegai2_DDP = term_omegai2_DDP + ( m * l * Mag2_omegai(i) * qi_inert(i).val );
    term_DOmega_DOmega = term_DOmega_DOmega + ( m * ri_skew(i).val * Ro' * qi_inert(i).val * qi_inert(i).val' * Ro * ri_skew(i).val );
    term_Omega2_DOmega = term_Omega2_DOmega + ( m * ri_skew(i).val * Ro' * qi_inert(i).val * qi_inert(i).val' * Ro * Omegao_skew * Omegao_skew * ri(i).val );
    term_omegai2_DOmega = term_omegai2_DOmega + ( m * l * ri_skew(i).val * Ro' * Mag2_omegai(i) * qi_inert(i).val );
    term_DDP_DOmega = term_DDP_DOmega + ( m * ri_skew(i).val * Ro' * qi_inert(i).val * qi_inert(i).val' );
    term_g_DOmega = term_g_DOmega + ( m * ri_skew(i).val * Ro' * qi_inert(i).val * qi_inert(i).val' * G );
    
    M_tot(6+(i-1)*3+1:6+(i-1)*3+3,1:3) = -1 * m * qi_inert_skew(i).val;
    M_tot(6+(i-1)*3+1:6+(i-1)*3+3,4:6) = m * qi_inert_skew(i).val * Ro * ri_skew(i).val;
    M_tot(6+(i-1)*3+1:6+(i-1)*3+3,6+(i-1)*3+1:6+(i-1)*3+3) = m * l * eye(3);
    
    F_tot(6+(i-1)*3+1:6+(i-1)*3+3,1) = ( m * qi_inert_skew(i).val * G ) + ( m * qi_inert_skew(i).val * Ro * Omegao_skew * Omegao_skew * ri(i).val ) - ...
        ( qi_inert_skew(i).val * Ui_local(i).val ); 
    
    D_Omega_Qi(i).val = (Jq ^ (-1)) * ( Mq(i).val - (Omega_Qi_skew(i).val * Jq * Omega_Qi(i).val) );
end

M_tot(1:3,1:3) = M * eye(3);
M_tot(1:3,4:6) = -1 * term_DOmega_DDP;

M_tot(4:6,1:3) = term_DDP_DOmega;
M_tot(4:6,4:6) = Jo - term_DOmega_DOmega;

F_tot(1:3,1) = u_DDP + term_g_DDP - term_omegai2_DDP - term_Omega2_DDP;
F_tot(4:6,1) = u_DOmega - term_g_DOmega - (Omegao_skew * Jo * Omegao) - term_omegai2_DOmega - term_Omega2_DOmega;

DX_tot = M_tot^(-1) * F_tot;

DD_Po = DX_tot(1:3,1);
D_Omegao = DX_tot(4:6,1);
D_omegai_1 = DX_tot(7:9,1);
D_omegai_2 = DX_tot(10:12,1);
D_omegai_3 = DX_tot(13:15,1);
D_omegai_4 = DX_tot(16:18,1);

D_Omega_Q1 = D_Omega_Qi(1).val;
D_Omega_Q2 = D_Omega_Qi(2).val;
D_Omega_Q3 = D_Omega_Qi(3).val;
D_Omega_Q4 = D_Omega_Qi(4).val;

%% Angles of links and their rates
omega1_skew = ...
    [0 -omegai1(3) omegai1(2);
    omegai1(3) 0 -omegai1(1);
    -omegai1(2) omegai1(1) 0];

omega2_skew = ...
    [0 -omegai2(3) omegai2(2);
    omegai2(3) 0 -omegai2(1);
    -omegai2(2) omegai2(1) 0];

omega3_skew = ...
    [0 -omegai3(3) omegai3(2);
    omegai3(3) 0 -omegai3(1);
    -omegai3(2) omegai3(1) 0];

omega4_skew = ...
    [0 -omegai4(3) omegai4(2);
    omegai4(3) 0 -omegai4(1);
    -omegai4(2) omegai4(1) 0];

Dq1 = omega1_skew * q1;
Dq2 = omega2_skew * q2;
Dq3 = omega3_skew * q3;
Dq4 = omega4_skew * q4;

Domega1_skew = ...
    [0 -D_omegai_1(3) D_omegai_1(2);
    D_omegai_1(3) 0 -D_omegai_1(1);
    -D_omegai_1(2) D_omegai_1(1) 0];

Domega2_skew = ...
    [0 -D_omegai_2(3) D_omegai_2(2);
    D_omegai_2(3) 0 -D_omegai_2(1);
    -D_omegai_2(2) D_omegai_2(1) 0];

Domega3_skew = ...
    [0 -D_omegai_3(3) D_omegai_3(2);
    D_omegai_3(3) 0 -D_omegai_3(1);
    -D_omegai_3(2) D_omegai_3(1) 0];

Domega4_skew = ...
    [0 -D_omegai_4(3) D_omegai_4(2);
    D_omegai_4(3) 0 -D_omegai_4(1);
    -D_omegai_4(2) D_omegai_4(1) 0];

DDq1 = Domega1_skew*q1 + omega1_skew*Dq1;
DDq2 = Domega2_skew*q2 + omega2_skew*Dq2;
DDq3 = Domega3_skew*q3 + omega3_skew*Dq3;
DDq4 = Domega4_skew*q4 + omega4_skew*Dq4;

%% Euler angles of the payload and their rates
R_f_o = [1 0 -sin(theta);
    0 cos(phi) cos(theta)*sin(phi);
    0 -sin(phi) cos(theta)*cos(phi)];

D_PHI = (R_f_o^-1) * Omegao;

DR_f_o = [0 0 -D_PHI(2)*cos(theta);
    0 -D_PHI(1)*sin(phi) (-D_PHI(2)*sin(theta)*sin(phi))+(D_PHI(1)*cos(theta)*cos(phi));
    0 -D_PHI(1)*cos(phi) (-D_PHI(2)*sin(theta)*cos(phi))-(D_PHI(1)*cos(theta)*sin(phi))];

DD_PHI = (R_f_o^-1) * ( D_Omegao - DR_f_o*D_PHI );

end

== matlab function Simple_4Quad_payload_04/Controllers and Observers/Controller and Observer - Agent2/Controller Interpreter #2 ==
  data: ut_2 input; PHI_d_2 output
function PHI_d_2 = fcn(ut_2)

%%
fT_2 = sqrt((ut_2(1)^2)+(ut_2(2)^2)+(ut_2(3)^2));
psi_d_2 = 0;
phi_d_2 = asin( min(max(((sin(psi_d_2)*ut_2(1) - cos(psi_d_2)*ut_2(2)) / (fT_2+1e-3)),-1),1) );
theta_d_2 = atan( (cos(psi_d_2)*ut_2(1) + sin(psi_d_2)*ut_2(2)) / (ut_2(3)+1e-3) );
PHI_d_2 = [phi_d_2;theta_d_2;psi_d_2]; 

end

== matlab function Simple_4Quad_payload_04/Controllers and Observers/Controlelr and Observer - Agent3/Controller Interpreter #3 ==
  data: ut_3 input; PHI_d_3 output
function PHI_d_3 = fcn(ut_3)

%%
fT_3 = sqrt((ut_3(1)^2)+(ut_3(2)^2)+(ut_3(3)^2));
psi_d_3 = 0;
phi_d_3 = asin( min(max(((sin(psi_d_3)*ut_3(1) - cos(psi_d_3)*ut_3(2)) / (fT_3+1e-3)),-1),1) );
theta_d_3 = atan( (cos(psi_d_3)*ut_3(1) + sin(psi_d_3)*ut_3(2)) / (ut_3(3)+1e-3) );
PHI_d_3 = [phi_d_3;theta_d_3;psi_d_3]; 

end

== matlab function Simple_4Quad_payload_04/Controllers and Observers/Controller and Observer - Agent2/Rotational #2/CARE ==
  data: P input; a_hat input; BR parameter; R parameter; DP output; QR parameter
function DP = fcn(P,a_hat,BR,R,QR)

DP = a_hat*P + P*a_hat' - P*BR*R*BR'*P + 2*QR;

end

== matlab function Simple_4Quad_payload_04/Controllers and Observers/Controller and Observer - Agent2/Rotational #2/Differentiator/Sliding differentiator ==
  data: u output; u1 input; e input; n parameter; k1 parameter
function u = fcn(u1,e,n,k1)

b=k1;

ABS = zeros(n,1);
for i=1:n
    if e(i)>0
        ABS(i) = e(i);
    else
        ABS(i) = -e(i);
    end
end
SGN = e ./ (ABS + 0.01);

u = u1 - b*(ABS.^0.5).*SGN;

end

== matlab function Simple_4Quad_payload_04/Controllers and Observers/Controller and Observer - Agent2/Rotation_Q2/D Phi ==
  data: Omega_Q2 input; D_PHI_Q2 output; PHI_Q2 input
function D_PHI_Q2 = fcn(Omega_Q2,PHI_Q2)

phi_q2 = PHI_Q2(1);
theta_q2 = PHI_Q2(2);

Rm_Q2 = [1 0 -sin(theta_q2);
    0 cos(phi_q2) cos(theta_q2)*sin(phi_q2);
    0 -sin(phi_q2) cos(theta_q2)*cos(phi_q2)];

D_PHI_Q2 = (Rm_Q2)^(-1) * Omega_Q2;


end

== matlab function Simple_4Quad_payload_04/Controllers and Observers/Controller and Observer - Agent2/Rotational #2/Differentiator/Sliding differentiator1 ==
  data: Du1 output; e input; n parameter; k2 parameter
function Du1 = fcn(e,n,k2)

a=k2;

ABS = zeros(n,1);
for i=1:n
    if e(i)>0
        ABS(i) = e(i);
    else
        ABS(i) = -e(i);
    end
end
SGN = e ./ (ABS + 0.01);

Du1 = - a*SGN;

end

== matlab function Simple_4Quad_payload_04/Controllers and Observers/Controller and Observer - Agent2/Rotational #2/g-Estimator ==
  data: sigma input; g_hat input; P input; rho_1 parameter; gamma_1 parameter; Dg_hat output
function Dg_hat = fcn(sigma,g_hat,P,rho_1,gamma_1)

Dg_hat = - gamma_1 * P * sigma - rho_1 * gamma_1 * g_hat;

end

== matlab function Simple_4Quad_payload_04/Controllers and Observers/Controller and Observer - Agent2/Rotational #2/g-Estimator1 ==
  data: sigma input; x input; P input; rho_0 parameter; gamma_0 parameter; Da_hat output; a_hat input
function Da_hat = fcn(sigma,x,P,rho_0,gamma_0,a_hat)

DVa_hat = - gamma_0 * P * diag(sigma) * (x - sigma) - rho_0 * gamma_0 * diag(a_hat);

Da_hat = diag(DVa_hat);

end

== matlab function Simple_4Quad_payload_04/Controllers and Observers/Controller and Observer - Agent2/Rotational #2/main ==
  data: sigma input; zeta input; u output; Dy_d input; R parameter; P input; a_hat input; BR parameter; g_hat input; x input; QR parameter; BBT_inv parameter; n parameter
function u = fcn(sigma,zeta,Dy_d,R,P,a_hat,BR,g_hat,x,QR,BBT_inv,n)

u1 = (1/2) * R * BR' * P * sigma;
u2 = BBT_inv * (Dy_d - a_hat*x + (eye(n) + 2*(((P)^(-1)*QR)) + a_hat)*sigma - g_hat - zeta) - (3/4) * R * BR' * P * sigma;

u = u1 + u2;

end

== matlab function Simple_4Quad_payload_04/Controllers and Observers/Controller and Observer - Agent2/Rotational #2/variable change ==
  data: X input; Xd input; x_mod output; u input; xd_mod output; e_mod output
function [x_mod,xd_mod,e_mod] = fcn(X,Xd,u)

x_mod = X;

xd_mod = [Xd;u(1:3)];

e_mod = xd_mod - x_mod;


end

== matlab function Simple_4Quad_payload_04/Controllers and Observers/Controlelr and Observer - Agent3/Rotation_Q3/D Phi ==
  data: Omega_Q3 input; D_PHI_Q3 output; PHI_Q3 input
function D_PHI_Q3 = fcn(Omega_Q3,PHI_Q3)

phi_q3 = PHI_Q3(1);
theta_q3 = PHI_Q3(2);

Rm_Q3 = [1 0 -sin(theta_q3);
    0 cos(phi_q3) cos(theta_q3)*sin(phi_q3);
    0 -sin(phi_q3) cos(theta_q3)*cos(phi_q3)];

D_PHI_Q3 = (Rm_Q3)^(-1) * Omega_Q3;


end

== matlab function Simple_4Quad_payload_04/Controllers and Observers/Controller and Observer - Agent4/Rotation_Q4/D Phi ==
  data: Omega_Q4 input; D_PHI_Q4 output; PHI_Q4 input
function D_PHI_Q4 = fcn(Omega_Q4,PHI_Q4)

phi_q4 = PHI_Q4(1);
theta_q4 = PHI_Q4(2);

Rm_Q4 = [1 0 -sin(theta_q4);
    0 cos(phi_q4) cos(theta_q4)*sin(phi_q4);
    0 -sin(phi_q4) cos(theta_q4)*cos(phi_q4)];

D_PHI_Q4 = (Rm_Q4)^(-1) * Omega_Q4;


end

== matlab function Simple_4Quad_payload_04/Dynamic model of the entire system/links angels computation ==
  data: q1 input; alphas output; betas output; Dalphas output; Dbetas output; q2 input; q3 input; q4 input; Dq1 input; Dq2 input; Dq3 input; Dq4 input
function [alphas,betas,Dalphas,Dbetas] = fcn(q1,q2,q3,q4,Dq1,Dq2,Dq3,Dq4)

alpha1 = asin(max(min(q1(3),1),-1));
beta1 = atan2(q1(2),q1(1));
if beta1 < (-3*pi/4)
    beta1 = 2*pi + beta1;
end
Dalpha1 = Dq1(3)/(cos(alpha1)+0.01);
Dbeta1 = ( Dq1(2)*cos(beta1) - Dq1(1)*sin(beta1) ) / (cos(alpha1)+0.01);



alpha2 = asin(max(min(q2(3),1),-1));
beta2 = atan2(q2(2),q2(1));
if beta2 < (-3*pi/4)
    beta2 = 2*pi + beta2;
end
Dalpha2 = Dq2(3)/(cos(alpha2)+0.01);
Dbeta2 = ( Dq2(2)*cos(beta2) - Dq2(1)*sin(beta2) ) / (cos(alpha2)+0.01);



alpha3 = asin(max(min(q3(3),1),-1));
beta3 = atan2(q3(2),q3(1));
if beta3 < (-3*pi/4)
    beta3 = 2*pi + beta3;
end
Dalpha3 = Dq3(3)/(cos(alpha3)+0.01);
Dbeta3 = ( Dq3(2)*cos(beta3) - Dq3(1)*sin(beta3) ) / (cos(alpha3)+0.01);



alpha4 = asin(max(min(q4(3),1),-1));
beta4 = atan2(q4(2),q4(1));
if beta4 < (-3*pi/4)
    beta4 = 2*pi + beta4;
end
Dalpha4 = Dq4(3)/(cos(alpha4)+0.01);
Dbeta4 = ( Dq4(2)*cos(beta4) - Dq4(1)*sin(beta4) ) / (cos(alpha4)+0.01);


alphas = [alpha1;alpha2;alpha3;alpha4];
betas = [beta1;beta2;beta3;beta4];
Dalphas = [Dalpha1;Dalpha2;Dalpha3;Dalpha4];
Dbetas = [Dbeta1;Dbeta2;Dbeta3;Dbeta4];

end

== matlab function Simple_4Quad_payload_04/Controllers and Observers/Controlelr and Observer - Agent3/Rotational #3/CARE ==
  data: P input; a_hat input; BR parameter; R parameter; DP output; QR parameter
function DP = fcn(P,a_hat,BR,R,QR)

DP = a_hat*P + P*a_hat' - P*BR*R*BR'*P + 2*QR;

end
